simulink model "16_Two_Lead_Sim"  (R2021a)
settings: Solver=VariableStepAuto  StartTime=0.0  StopTime=10.0  RelTol=1e-3
settings Model: Creator=ideapad  LastModifiedBy=ideapad

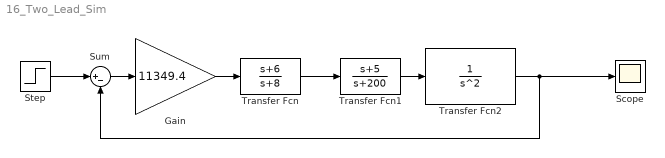
== system 16_Two_Lead_Sim ==
  Gain : Gain  Gain=11349.4
  Scope : Scope
  Step : Step  SampleTime=0
  Sum : Sum  Inputs=|+-
  Transfer Fcn : TransferFcn  Numerator=[1 6]  Denominator=[1 8]
  Transfer Fcn1 : TransferFcn  Numerator=[1 5]  Denominator=[1 200]
  Transfer Fcn2 : TransferFcn  Denominator=[1 0 0]
  wires:
  Gain/1 -> Transfer Fcn/1
  Transfer Fcn/1 -> Transfer Fcn1/1
  Sum/1 -> Gain/1
  Step/1 -> Sum/1
  Transfer Fcn1/1 -> Transfer Fcn2/1
  Transfer Fcn2/1 -> Scope/1, Sum/2
